simulink library "slrtresolverlib"  (R2022a)
settings: Solver=VariableStepAuto  StartTime=0.0  StopTime=10.0  RelTol=1e-3
libraries: simulink x1, hdlsllib x1
settings Model: Creator=chrisz  LastModifiedBy=chrisz

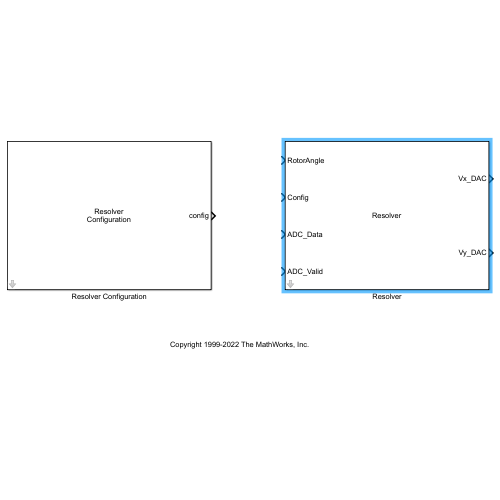
[thumbnail: Simulink's stored preview of the top-level diagram]
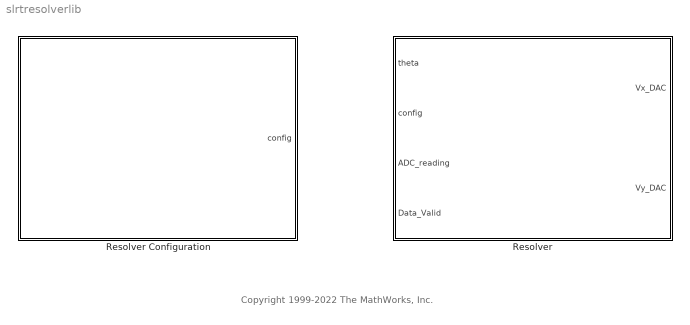
== system slrtresolverlib ==
  note: Copyright 1999-2022 The MathWorks, Inc.
  Resolver : Subsystem  mask(Resolveer){Ts=1e-6}
      mask prompts: Ts "Sample time (s):"
      mask help: HDL coder compatible implementation of resolver. This model simulates FPGA clock level operations and is not suited for desktop simulation other than for validating the real-time model is accurate. It should primarily be used when generating HDL for real-time systems. Use standard blocks for desktop simulation.
      mask Display:
      | disp('Resolver')
      | port_label('input', 1, 'RotorAngle')
      | port_label('input', 2, 'Config')
      | port_label('input', 3, 'ADC_Data')
      | port_label('input', 4, 'ADC_Valid')
      | port_label('output', 1, 'Vx_DAC')
      | port_label('output', 2, 'Vy_DAC')
  Resolver Configuration : Subsystem  mask(Resolver Configuration){Ts=1e-6, R=0.5, N=1, ADCrefV=5, ADCbits=12, totalADCCounts=4096}
      mask prompts: Ts "Sample time (s)"; R "Transformation ratio"; N "Number of pole pairs"; ADCrefV "ADC reference voltage (V):"; ADCbits "ADC number of bits:"
      mask help: Configuration block for HDL coder compatible implementation of resolver. This block intends to be used for configuaring the corresponding resolver block on FPGA.
      mask Callback ADCbits:
      | mask = Simulink.Mask.get(gcb);
      | ADCbits = str2num(get_param(gcb,'ADCbits'));
      | mask.getParameter('totalADCCounts').Value = num2str(2^ADCbits);
      mask DialogControl Container3 Prompt: Block options
      mask Display:
      | disp('Resolver\nConfiguration');
      | port_label('output', 1, 'config')

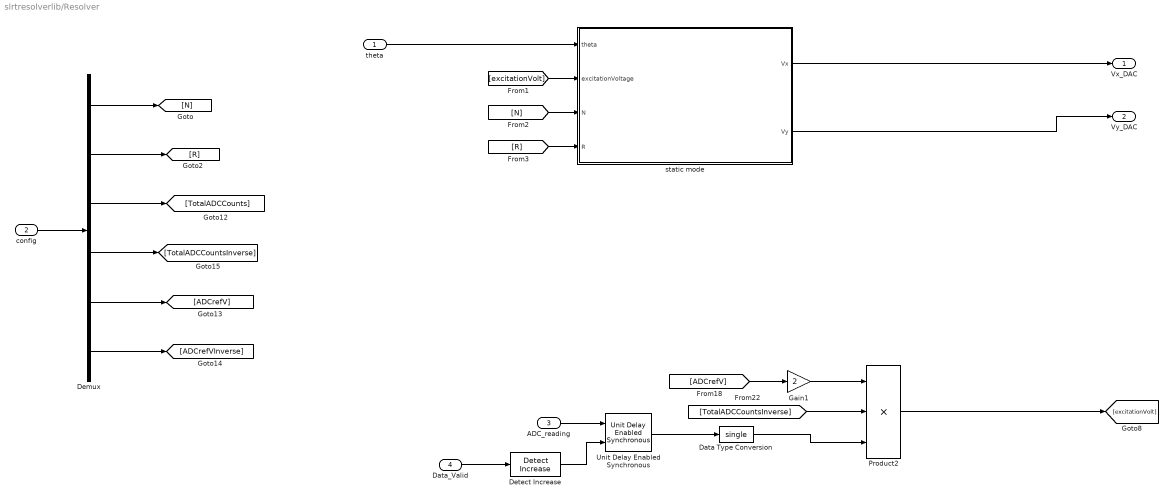
== system slrtresolverlib/Resolver ==
  theta : Inport
  config : Inport  Port=2
  ADC_reading : Inport  Port=3
  Data_Valid : Inport  Port=4
  Data Type Conversion : DataTypeConversion  OutDataTypeStr=single  SaturateOnIntegerOverflow=off  RndMeth=Floor
  Demux : Demux  Outputs=6
  Detect Increase : simulink/Logic and Bit Operations/Detect Increase  vinit=0.0  OutDataTypeStr=boolean
  Gain1 : Gain  Gain=2
  Product2 : Product  Inputs=3
  Unit Delay Enabled Synchronous : hdlsllib/Discrete/Unit Delay Enabled Synchronous  InitialCondition=0.0  SampleTime=-1
      settings: SourceProductBaseCode=SL
  static mode : Subsystem  TreatAsAtomicUnit=on
  Vx_DAC : Outport
  Vy_DAC : Outport  Port=2
  wires:
  config/1 -> Demux/1
  theta/1 -> static mode/1(theta)
  [excitationVolt] -> static mode/2(excitationVoltage)
  [N] -> static mode/3(N)
  [R] -> static mode/4(R)
  Product2/1 -> [excitationVolt]
  [ADCrefV] -> Gain1/1
  Gain1/1 -> Product2/1
  [TotalADCCountsInverse] -> Product2/2
  Data Type Conversion/1 -> Product2/3
  Data_Valid/1 -> Detect Increase/1
  Detect Increase/1 -> Unit Delay Enabled Synchronous/2
  ADC_reading/1 -> Unit Delay Enabled Synchronous/1
  Unit Delay Enabled Synchronous/1 -> Data Type Conversion/1
  static mode/1(Vx) -> Vx_DAC/1
  static mode/2(Vy) -> Vy_DAC/1
  Demux/3 -> [TotalADCCounts]
  Demux/2 -> [R]
  Demux/1 -> [N]
  Demux/4 -> [TotalADCCountsInverse]
  Demux/5 -> [ADCrefV]
  Demux/6 -> [ADCrefVInverse]

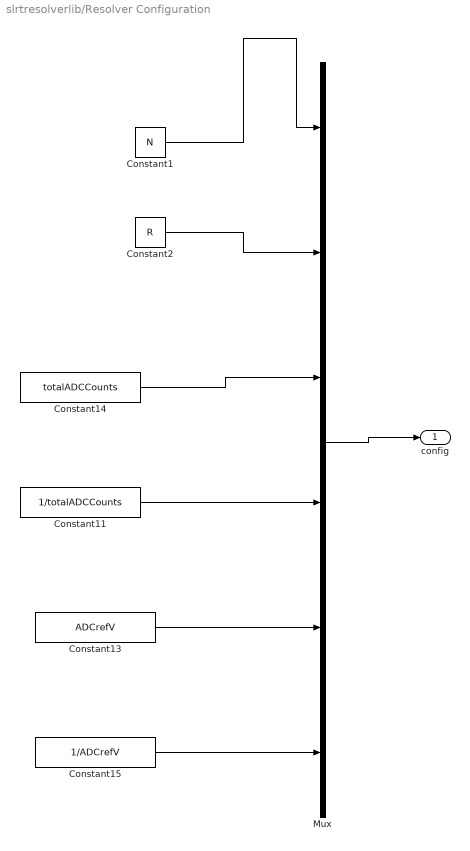
== system slrtresolverlib/Resolver Configuration ==
  Constant1 : Constant  Value=N  OutDataTypeStr=single  SampleTime=Ts
  Constant11 : Constant  Value=1/totalADCCounts  OutDataTypeStr=single  SampleTime=Ts
  Constant13 : Constant  Value=ADCrefV  OutDataTypeStr=single  SampleTime=Ts
  Constant14 : Constant  Value=totalADCCounts  OutDataTypeStr=single  SampleTime=Ts
  Constant15 : Constant  Value=1/ADCrefV  OutDataTypeStr=single  SampleTime=Ts
  Constant2 : Constant  Value=R  OutDataTypeStr=single  SampleTime=Ts
  Mux : Mux  Inputs=6
  config : Outport
  wires:
  Mux/1 -> config/1
  Constant14/1 -> Mux/3
  Constant11/1 -> Mux/4
  Constant13/1 -> Mux/5
  Constant15/1 -> Mux/6
  Constant1/1 -> Mux/1
  Constant2/1 -> Mux/2

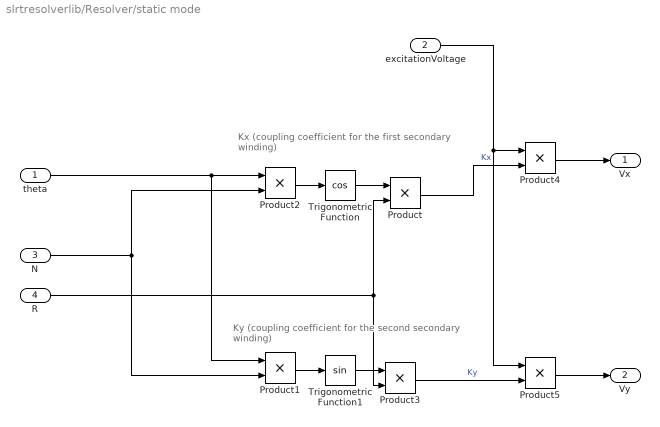
== system slrtresolverlib/Resolver/static mode ==
  note: Ky (coupling coefficient for the second
      | secondary winding)
  note: Kx (coupling coefficient for the first
      | secondary winding)
  theta : Inport
  excitationVoltage : Inport  Port=2
  N : Inport  Port=3
  R : Inport  Port=4
  Product{,1..5} (6 alike) : Product
  Trigonometric Function : Trigonometry  Operator=cos
  Trigonometric Function1 : Trigonometry
  Vx : Outport  InitialOutput=0
  Vy : Outport  Port=2  InitialOutput=0
  wires:
  Product4/1 -> Vx/1
  Product5/1 -> Vy/1
  Trigonometric Function1/1 -> Product3/1
  excitationVoltage/1 -> Product5/1, Product4/1
  Trigonometric Function/1 -> Product/1
  Product/1 -> Product4/2  "Kx"
  Product3/1 -> Product5/2  "Ky"
  Product2/1 -> Trigonometric Function/1
  Product1/1 -> Trigonometric Function1/1
  theta/1 -> Product1/1, Product2/1
  N/1 -> Product1/2, Product2/2
  R/1 -> Product/2, Product3/2
